simulink model "ROS_3_20"  (R2021b)
settings: Solver=VariableStepAuto  StartTime=0.0  StopTime=inf  RelTol=1e-3
undefined symbols (not defined in the file): X, Y
libraries: robotlib x4
settings Model: Creator=FOR  LastModifiedBy=FOR

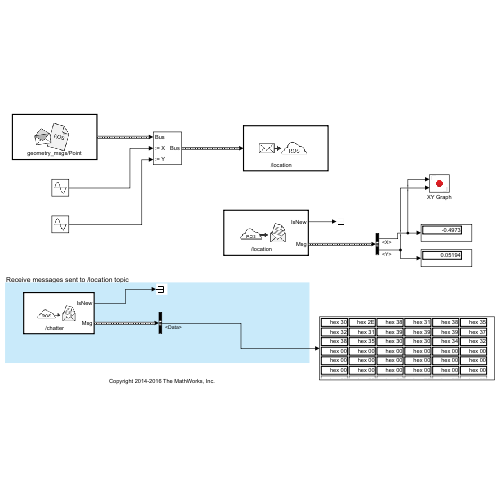
[thumbnail: Simulink's stored preview of the top-level diagram]
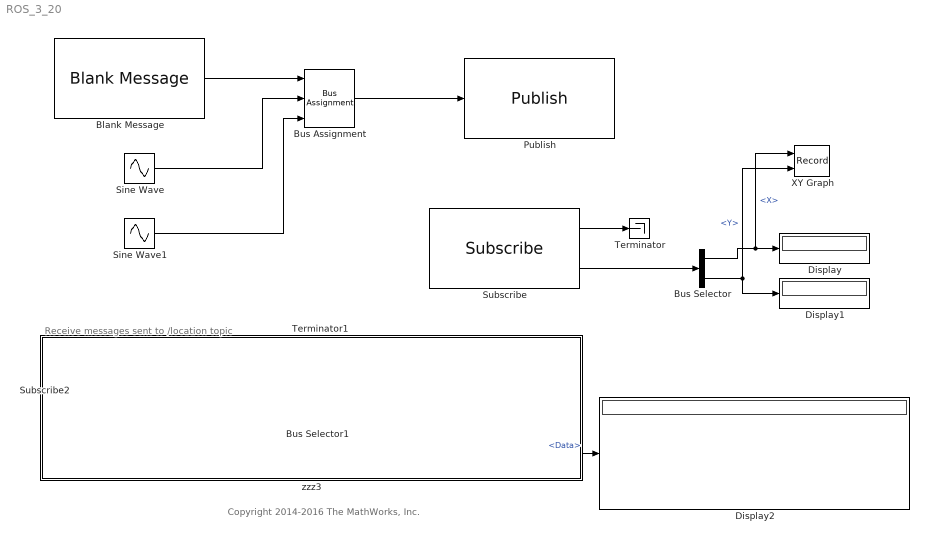
== system ROS_3_20 ==
  note: Receive messages sent to /location topic
  note: Copyright 2014-2016 The MathWorks, Inc.
  Blank Message : robotlib/Blank Message  messageClass=Message  entityType=geometry_msgs/Point  messageType=geometry_msgs/Point  SampleTime=inf  legacyBusStruct=off
  Bus Assignment : BusAssignment  AssignedSignals=X,Y
  Bus Selector : BusSelector  OutputSignals=X,Y
  Bus Selector1 : BusSelector  OutputSignals=Data
  Display : Display
  Display1 : Display
  Display2 : Display
      settings: Format=hex (Stored Integer)
  Publish : robotlib/Publish  topicSource=Specify your own  topic=/location  messageType=geometry_msgs/Point  legacyBusStruct=off  messageQueueLength=1
  Sine Wave : Sin  Amplitude=0.5  SampleTime=0
  Sine Wave1 : Sin  Amplitude=0.5  Phase=pi/2  SampleTime=0
  Subscribe : robotlib/Subscribe  topicSource=Specify your own  topic=/location  messageType=geometry_msgs/Point  SampleTime=-1  legacyBusStruct=off  messageQueueLength=1
  Subscribe2 : robotlib/Subscribe  topicSource=Specify your own  topic=/chatter  messageType=std_msgs/String  SampleTime=-1  legacyBusStruct=off  messageQueueLength=51
  Terminator : Terminator
  Terminator1 : Terminator
  XY Graph : Record  FileSettingsInternal="{\"entries\":[{\"content\":{\"excelSettings\":{\"content\":{},\"type\":\"Streamout.ExcelSettings\"}},\"type\":\"Streamout.FileSettingStorage\",\"uuid\":\"d1619efe-be70-4b63-9b89-2ce50da9c412\"}],\"packageUris\":[\"http://schema.mathworks.com/mf0/streamout_blocks/R2020a\"],\"version\":\"1.0\"}"  Layout=[1 1]  SignalsInternal="{\"entries\":[{\"content\":{\"signals\":[{\"content\":{\"blockPath\":[\"ROS_3_20/XY Graph\"],\"channel\":[],\"dimensions\":[1],\"domain\":\"ROS_3_20/XY Graph\",\"lineColor\":\"#a2142f\",\"plots\":[1],\"port\":1,\"sid\":[\"\"],\"signalID\":26086,\"signalName\":\"<X>\"},\"type\":\"RecordBlkView.Signal\",\"uuid\":\"0d8cbf0a-c267-4b30-9f85-e7bdbf8ad0dc\"},{\"content\":{\"blockPath\":[\"ROS_3_20/XY Graph\"],\"channel\":[],\"dimensions\":[1],\"domain\":\"ROS_3_20/XY Graph\",\"lineColor\":\"#139fff\",\"plots\":[1],\"port\":2,\"sid\":[\"\"],\"signalID\":26090,\"signalName\":\"<Y>\"},\"type\":\"RecordBlkView.Signal\",\"uuid\":\"137285f0-6821-4f97-a17d-da7db499d01a\"}]},\"type\":\"RecordBlkView.InputSignals\",\"uuid\":\"ed7015e3-edb0-48f9-90ae-a3910abe0220\"}],\"packageUris\":[\"http://schema.mathworks.com/mf0/streamout_blocks/R2020a\"],\"version\":\"1.0\"}"  VisualizationBindings="{\"xyplotplugin\":{\"info\":[{\"series\":[{\"bindingParametersList\":[{\"parameter\":\"X-Axis\",\"signalID\":26086,\"signalName\":\"<X>\"},{\"parameter\":\"Y-Axis\",\"signalID\":26090,\"signalName\":\"<Y>\"}],\"seriesID\":64864}],\"subplotID\":1}]}}"  CompatibilityTag=XY
  zzz3 : Subsystem  TreatAsAtomicUnit=on
      settings: OpenFcn=% no-op
      mask Display: disp('')
  wires:
  Blank Message/1 -> Bus Assignment/1
  Sine Wave/1 -> Bus Assignment/2
  Sine Wave1/1 -> Bus Assignment/3
  Bus Assignment/1 -> Publish/1
  Subscribe/2 -> Bus Selector/1
  Bus Selector/1 -> XY Graph/1, Display/1  "<X>"
  Bus Selector/2 -> XY Graph/2, Display1/1  "<Y>"
  Subscribe/1 -> Terminator/1
  Bus Selector1/1 -> Display2/1  "<Data>"
  Subscribe2/1 -> Terminator1/1
  Subscribe2/2 -> Bus Selector1/1

== system ROS_3_20/zzz3 ==
